simulink model "GitEntegrasyon"  (R2022a)
settings: Solver=VariableStepAuto  StartTime=0.0  StopTime=10.0  RelTol=1e-3
libraries: simulink x8, AIOS_Lib x1
settings Model: Creator=ISU30922  LastModifiedBy=ISU30922

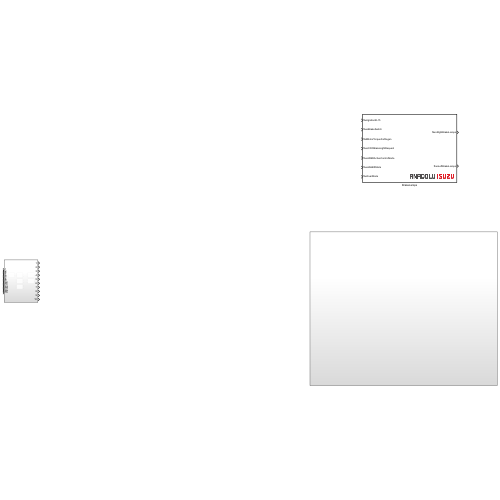
[thumbnail: Simulink's stored preview of the top-level diagram]
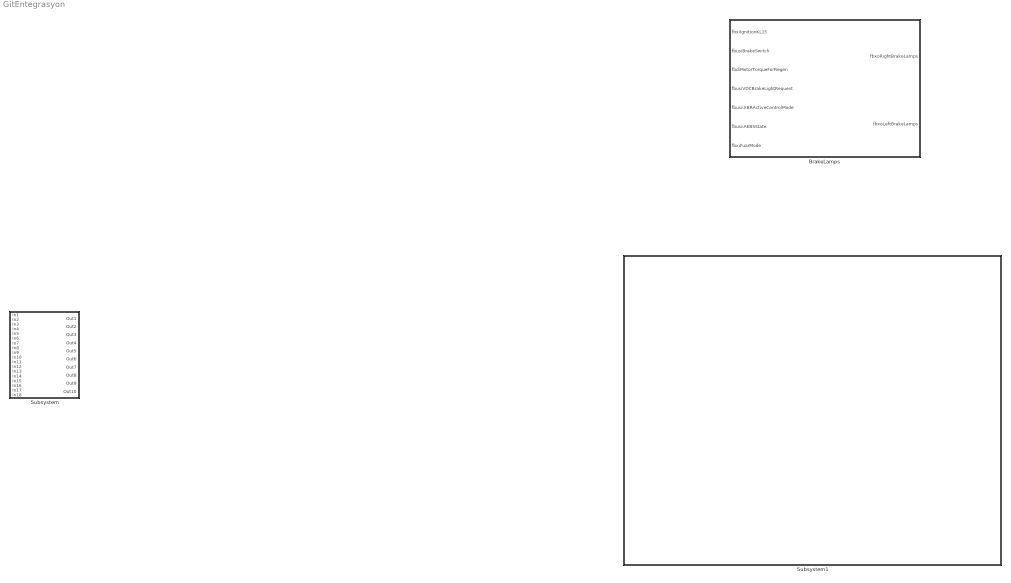
== system GitEntegrasyon ==
  BrakeLamps : Subsystem  TreatAsAtomicUnit=on
      mask Display: image('$imagefile'); % Use "Edit Image" on toolstrip to change.
  Subsystem : Subsystem
  Subsystem1 : Subsystem

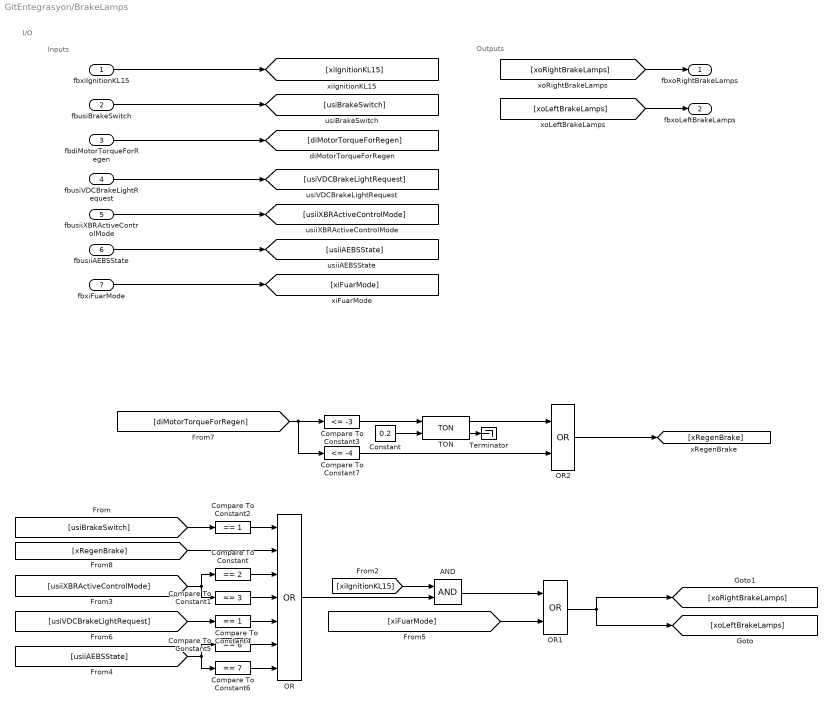
== system GitEntegrasyon/BrakeLamps ==
  note: I/O
  note: Outputs
  note: Inputs
  fbxiIgnitionKL15 : Inport  OutDataTypeStr=boolean
  fbusiBrakeSwitch : Inport  Port=2  OutDataTypeStr=uint8
  fbdiMotorTorqueForRegen : Inport  Port=3  OutDataTypeStr=double
  fbusiVDCBrakeLightRequest : Inport  Port=4  OutDataTypeStr=uint8
  fbusiiXBRActiveControlMode : Inport  Port=5  OutDataTypeStr=uint8
  fbusiiAEBSState : Inport  Port=6  OutDataTypeStr=uint8
  fbxiFuarMode : Inport  Port=7  OutDataTypeStr=boolean
  AND : Logic  AllPortsSameDT=off  OutDataTypeStr=boolean
  Compare To Constant : simulink/Logic and Bit Operations/Compare To Constant  relop===  const=2  OutDataTypeStr=boolean
  Compare To Constant1 : simulink/Logic and Bit Operations/Compare To Constant  relop===  const=3  OutDataTypeStr=boolean
  Compare To Constant2 : simulink/Logic and Bit Operations/Compare To Constant  relop===  const=1  OutDataTypeStr=boolean
  Compare To Constant3 : simulink/Logic and Bit Operations/Compare To Constant  relop=<=  const=-3  OutDataTypeStr=boolean
  Compare To Constant4 : simulink/Logic and Bit Operations/Compare To Constant  relop===  const=1  OutDataTypeStr=boolean
  Compare To Constant5 : simulink/Logic and Bit Operations/Compare To Constant  relop===  const=6  OutDataTypeStr=boolean
  Compare To Constant6 : simulink/Logic and Bit Operations/Compare To Constant  relop===  const=7  OutDataTypeStr=boolean
  Compare To Constant7 : simulink/Logic and Bit Operations/Compare To Constant  relop=<=  const=-4  OutDataTypeStr=boolean
  Constant : Constant  Value=0.2  OutDataTypeStr=single
  OR : Logic  Operator=OR  Inputs=7  AllPortsSameDT=off  OutDataTypeStr=boolean
  OR1 : Logic  Operator=OR  AllPortsSameDT=off  OutDataTypeStr=boolean
  OR2 : Logic  Operator=OR  AllPortsSameDT=off  OutDataTypeStr=boolean
  TON : AIOS_Lib/Standart Functions/TON  SystemSampleTime=-1  VariantActivationTime=update diagram  Latency=0  AutoFrameSizeCalculation=off
      settings: SourceProductName=AIOS Lib
  Terminator : Terminator
  fbxoRightBrakeLamps : Outport  OutDataTypeStr=boolean  VectorParamsAs1DForOutWhenUnconnected=off
  fbxoLeftBrakeLamps : Outport  Port=2  OutDataTypeStr=boolean  VectorParamsAs1DForOutWhenUnconnected=off
  wires:
  Compare To Constant6/1 -> OR/7
  Compare To Constant5/1 -> OR/6
  Compare To Constant4/1 -> OR/5
  [usiiAEBSState] -> Compare To Constant5/1, Compare To Constant6/1
  [usiVDCBrakeLightRequest] -> Compare To Constant4/1
  fbusiVDCBrakeLightRequest/1 -> [usiVDCBrakeLightRequest]
  [xRegenBrake] -> OR/2
  [usiBrakeSwitch] -> Compare To Constant2/1
  [xoRightBrakeLamps] -> fbxoRightBrakeLamps/1
  fbxiIgnitionKL15/1 -> [xiIgnitionKL15]
  fbusiBrakeSwitch/1 -> [usiBrakeSwitch]
  fbdiMotorTorqueForRegen/1 -> [diMotorTorqueForRegen]
  fbusiiXBRActiveControlMode/1 -> [usiiXBRActiveControlMode]
  fbusiiAEBSState/1 -> [usiiAEBSState]
  Compare To Constant2/1 -> OR/1
  OR/1 -> AND/2
  [xiIgnitionKL15] -> AND/1
  OR1/1 -> [xoLeftBrakeLamps], [xoRightBrakeLamps]
  [usiiXBRActiveControlMode] -> Compare To Constant/1, Compare To Constant1/1
  Compare To Constant/1 -> OR/3
  Compare To Constant1/1 -> OR/4
  [xoLeftBrakeLamps] -> fbxoLeftBrakeLamps/1
  fbxiFuarMode/1 -> [xiFuarMode]
  AND/1 -> OR1/1
  [xiFuarMode] -> OR1/2
  [diMotorTorqueForRegen] -> Compare To Constant7/1, Compare To Constant3/1
  Compare To Constant3/1 -> TON/1
  Constant/1 -> TON/2
  TON/2 -> Terminator/1
  TON/1 -> OR2/1
  OR2/1 -> [xRegenBrake]
  Compare To Constant7/1 -> OR2/2

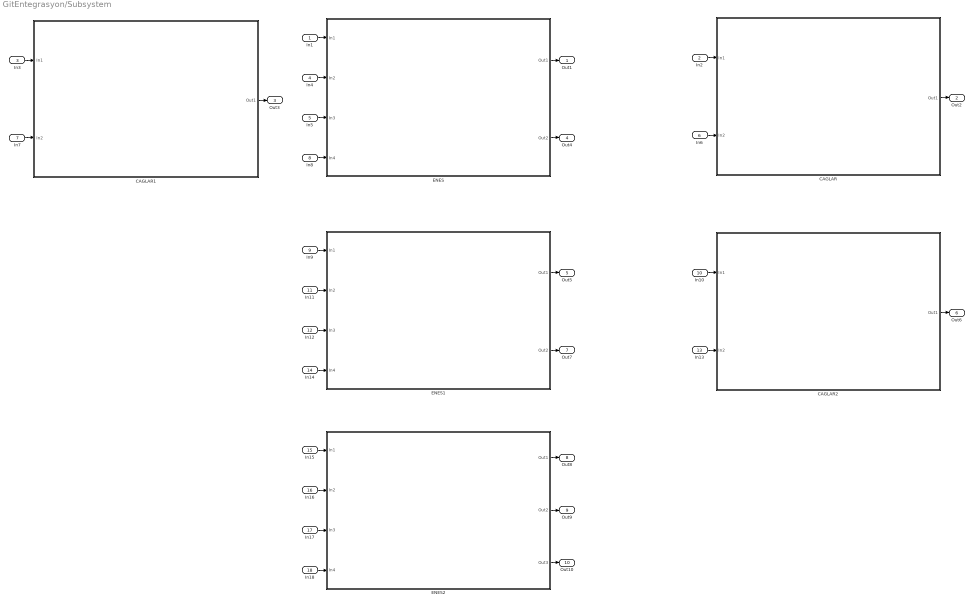
== system GitEntegrasyon/Subsystem ==
  In1 : Inport
  In2 : Inport  Port=2
  In3 : Inport  Port=3
  In4 : Inport  Port=4
  In5 : Inport  Port=5
  In6 : Inport  Port=6
  In7 : Inport  Port=7
  In8 : Inport  Port=8
  In9 : Inport  Port=9
  In10 : Inport  Port=10
  In11 : Inport  Port=11
  In12 : Inport  Port=12
  In13 : Inport  Port=13
  In14 : Inport  Port=14
  In15 : Inport  Port=15
  In16 : Inport  Port=16
  In17 : Inport  Port=17
  In18 : Inport  Port=18
  CAGLAR : Subsystem
  CAGLAR1 : Subsystem
  CAGLAR2 : Subsystem
  ENES : Subsystem
  ENES1 : Subsystem
  ENES2 : Subsystem
  Out1 : Outport
  Out2 : Outport  Port=2
  Out3 : Outport  Port=3
  Out4 : Outport  Port=4
  Out5 : Outport  Port=5
  Out6 : Outport  Port=6
  Out7 : Outport  Port=7
  Out8 : Outport  Port=8
  Out9 : Outport  Port=9
  Out10 : Outport  Port=10
  wires:
  In16/1 -> ENES2/2(In2)
  ENES2/3(Out3) -> Out10/1
  ENES/2(Out2) -> Out4/1
  CAGLAR/1(Out1) -> Out2/1
  In2/1 -> CAGLAR/1(In1)
  CAGLAR2/1(Out1) -> Out6/1
  In8/1 -> ENES/4(In4)
  In13/1 -> CAGLAR2/2(In2)
  ENES1/2(Out2) -> Out7/1
  In10/1 -> CAGLAR2/1(In1)
  In6/1 -> CAGLAR/2(In2)
  In1/1 -> ENES/1(In1)
  In17/1 -> ENES2/3(In3)
  In15/1 -> ENES2/1(In1)
  ENES/1(Out1) -> Out1/1
  In4/1 -> ENES/2(In2)
  In5/1 -> ENES/3(In3)
  CAGLAR1/1(Out1) -> Out3/1
  In12/1 -> ENES1/3(In3)
  In18/1 -> ENES2/4(In4)
  In7/1 -> CAGLAR1/2(In2)
  ENES1/1(Out1) -> Out5/1
  ENES2/2(Out2) -> Out9/1
  ENES2/1(Out1) -> Out8/1
  In11/1 -> ENES1/2(In2)
  In9/1 -> ENES1/1(In1)
  In3/1 -> CAGLAR1/1(In1)
  In14/1 -> ENES1/4(In4)

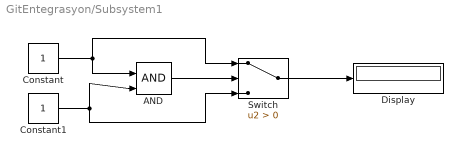
== system GitEntegrasyon/Subsystem1 ==
  AND : Logic  IconShape=distinctive  AllPortsSameDT=off  OutDataTypeStr=boolean
  Constant : Constant
  Constant1 : Constant
  Display : Display
  Switch : Switch  Criteria=u2 > Threshold  SaturateOnIntegerOverflow=off  InputSameDT=off
  wires:
  Constant/1 -> Switch/1, AND/1
  Constant1/1 -> Switch/3, AND/2
  AND/1 -> Switch/2
  Switch/1 -> Display/1

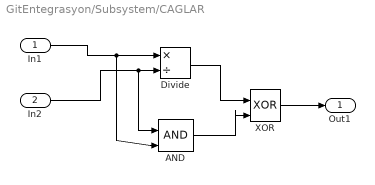
== system GitEntegrasyon/Subsystem/CAGLAR ==
  In1 : Inport
  In2 : Inport  Port=2
  AND : Logic  IconShape=distinctive  AllPortsSameDT=off  OutDataTypeStr=boolean
  Divide : Product  Inputs=*/
  XOR : Logic  Operator=XOR  IconShape=distinctive  AllPortsSameDT=off  OutDataTypeStr=boolean
  Out1 : Outport
  wires:
  In1/1 -> AND/2, Divide/1
  In2/1 -> AND/1, Divide/2
  Divide/1 -> XOR/1
  AND/1 -> XOR/2
  XOR/1 -> Out1/1

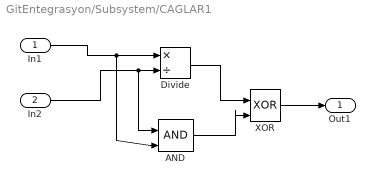
== system GitEntegrasyon/Subsystem/CAGLAR1 ==
  In1 : Inport
  In2 : Inport  Port=2
  AND : Logic  IconShape=distinctive  AllPortsSameDT=off  OutDataTypeStr=boolean
  Divide : Product  Inputs=*/
  XOR : Logic  Operator=XOR  IconShape=distinctive  AllPortsSameDT=off  OutDataTypeStr=boolean
  Out1 : Outport
  wires:
  In1/1 -> AND/2, Divide/1
  In2/1 -> AND/1, Divide/2
  Divide/1 -> XOR/1
  AND/1 -> XOR/2
  XOR/1 -> Out1/1

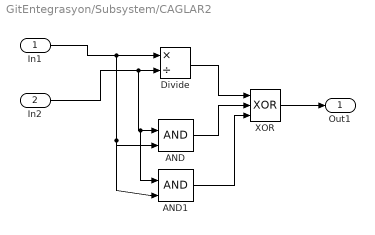
== system GitEntegrasyon/Subsystem/CAGLAR2 ==
  In1 : Inport
  In2 : Inport  Port=2
  AND : Logic  IconShape=distinctive  AllPortsSameDT=off  OutDataTypeStr=boolean
  AND1 : Logic  IconShape=distinctive  AllPortsSameDT=off  OutDataTypeStr=boolean
  Divide : Product  Inputs=*/
  XOR : Logic  Operator=XOR  Inputs=3  IconShape=distinctive  AllPortsSameDT=off  OutDataTypeStr=boolean
  Out1 : Outport
  wires:
  AND1/1 -> XOR/3
  In1/1 -> AND/2, AND1/2, Divide/1
  In2/1 -> AND/1, AND1/1, Divide/2
  Divide/1 -> XOR/1
  AND/1 -> XOR/2
  XOR/1 -> Out1/1

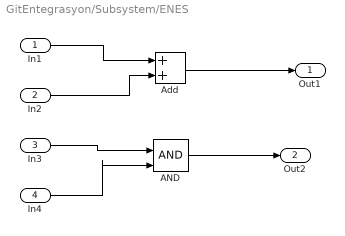
== system GitEntegrasyon/Subsystem/ENES ==
  In1 : Inport
  In2 : Inport  Port=2
  In3 : Inport  Port=3
  In4 : Inport  Port=4
  AND : Logic  IconShape=distinctive  AllPortsSameDT=off  OutDataTypeStr=boolean
  Add : Sum
  Out1 : Outport
  Out2 : Outport  Port=2
  wires:
  In1/1 -> Add/1
  In2/1 -> Add/2
  Add/1 -> Out1/1
  In3/1 -> AND/1
  In4/1 -> AND/2
  AND/1 -> Out2/1

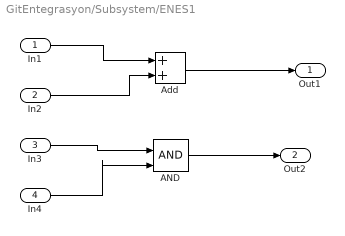
== system GitEntegrasyon/Subsystem/ENES1 ==
  In1 : Inport
  In2 : Inport  Port=2
  In3 : Inport  Port=3
  In4 : Inport  Port=4
  AND : Logic  IconShape=distinctive  AllPortsSameDT=off  OutDataTypeStr=boolean
  Add : Sum
  Out1 : Outport
  Out2 : Outport  Port=2
  wires:
  AND/1 -> Out2/1
  In4/1 -> AND/2
  In3/1 -> AND/1
  Add/1 -> Out1/1
  In2/1 -> Add/2
  In1/1 -> Add/1

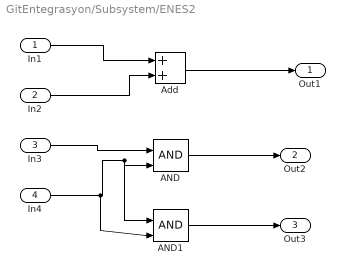
== system GitEntegrasyon/Subsystem/ENES2 ==
  In1 : Inport
  In2 : Inport  Port=2
  In3 : Inport  Port=3
  In4 : Inport  Port=4
  AND : Logic  IconShape=distinctive  AllPortsSameDT=off  OutDataTypeStr=boolean
  AND1 : Logic  IconShape=distinctive  AllPortsSameDT=off  OutDataTypeStr=boolean
  Add : Sum
  Out1 : Outport
  Out2 : Outport  Port=2
  Out3 : Outport  Port=3
  wires:
  In1/1 -> Add/1
  In2/1 -> Add/2
  Add/1 -> Out1/1
  In3/1 -> AND/1
  In4/1 -> AND1/2, AND1/1, AND/2
  AND/1 -> Out2/1
  AND1/1 -> Out3/1
